simulink model "boostObserver_old"  (R2020a)
settings: Solver=VariableStepAuto  StartTime=0.0  StopTime=3.2  FixedStep=0.0005  MaxStep=9e-06  RelTol=1e-03  EnableMultiTasking=on
InitFcn:
  | kp=0.01;
  | ki=0.01;
  | 
  | k=2;
  | em=100000000;
  | GE=1/em;
  | GU=k*ki/GE;
  | GCE=k*kp/GU;
model workspace (MAT data in the model file):
  time = 0.8
values from neighbouring files (symbols this model uses):
  A1 = obj.boostConverter.A1    [BoostController.m]    (also in BoostConverter.m = [-obj.R/obj.L 0;0 -1/(obj.Ro*obj.C)]; BuckBoostConverter.m = [-obj.R/obj.L 0;0 -1/(obj.Ro*obj.C)]; obsmc.m = Asigma{1,1}; workspace_atual.mat = [-16.4  0; 0  -3.50877192982])
  A2 = obj.boostConverter.A2    [BoostController.m]    (also in BoostConverter.m = [-obj.R/obj.L -1/obj.L;1/obj.C -1/(obj.Ro*obj.C)]; BuckBoostConverter.m = [-obj.R/obj.L 1/obj.L;-1/obj.C -1/(obj.Ro*obj.C)]; obsmc.m = Asigma{1,2}; workspace_atual.mat = [-16.4  -200; 350.877192982  -3.50877192982])
  AlarmDeadTime = 0.50    (= 0.5)    [BoostFaultSimulation.m]    (also in workspace_atual.mat; workspace_certo.mat)
  B1 = obj.boostConverter.B1    [BoostController.m]    (also in BoostConverter.m = [1/obj.L;0]; BuckBoostConverter.m = [1/obj.L;0]; obsmc.m = Bsigma{1,1}; workspace_atual.mat = [200 0])
  boost_parameters = [obj.Ro,obj.R,obj.L,obj.C,obj.u]'    [BoostConverter.m]    (also in BuckBoostConverter.m; boostResults2Latex.m = boost.parameters(); workspace_atual.mat = [100 0.082 0.005 0.00285 190]; workspace_certo.mat = [100 0.082 0.005 0.00285 190])
  C = 1e-3    (= 0.001)    [boostResults2Latex.m]
  CiL = [0 1]    [workspace_atual.mat]    (also in workspace_certo.mat)
  Cmatrix = [1  0; 0  1]    [workspace_atual.mat]    (also in workspace_certo.mat)
  CVc = [1 0]    [workspace_atual.mat]    (also in workspace_certo.mat)
  D1 = [1  0; 0  1]    [workspace_atual.mat]    (also in workspace_certo.mat)
  FaultClass = 0    [BoostFaultSimulation.m]    (also in workspace_atual.mat = 1; workspace_certo.mat = 1)
  iLFaultSwitch = 0    [BoostFaultSimulation.m]    (also in workspace_atual.mat; workspace_certo.mat)
  iLFaultTime = 1.70    (= 1.7)    [BoostFaultSimulation.m]    (also in workspace_atual.mat; workspace_certo.mat)
  iLGainFaultFactor = 15    [BoostFaultSimulation.m]    (also in workspace_atual.mat; workspace_certo.mat)
  iLNoiseFaultSwitch = 0    [BoostFaultSimulation.m]    (also in workspace_atual.mat; workspace_certo.mat)
  iLNoiseTime = 1.70    (= 1.7)    [BoostFaultSimulation.m]    (also in workspace_atual.mat; workspace_certo.mat)
  Jth = 2000    [workspace_atual.mat]    (also in workspace_certo.mat)
  L = 1e-3    (= 0.001)    [boostResults2Latex.m]    (also in obsmc.m = sdpvar(3,1,'full'))
  LoadAddResistor = obj.LoadAddFactor*obj.Ro    [BoostFaultSimulation.m]    (also in workspace_atual.mat = 30; workspace_certo.mat = 30)
  LoadAddSignalSwitch = 1    [BoostFaultSimulation.m]    (also in workspace_atual.mat; workspace_certo.mat)
  LoadAddSwitch = 0    [BoostFaultSimulation.m]    (also in workspace_atual.mat; workspace_certo.mat)
  LoadAddTime = 0.90    (= 0.9)    [BoostFaultSimulation.m]    (also in workspace_atual.mat; workspace_certo.mat)
  LoadRemoveResistor = obj.Ro*(1-obj.LoadRemoveFactor)/(obj.LoadRemoveFactor)    [BoostFaultSimulation.m]    (also in workspace_atual.mat = 233.333333333; workspace_certo.mat = 233.333333333)
  LoadRemoveSignalSwitch = 1    [BoostFaultSimulation.m]    (also in workspace_atual.mat; workspace_certo.mat)
  LoadRemoveSwitch = 0    [BoostFaultSimulation.m]    (also in workspace_atual.mat; workspace_certo.mat)
  LoadRemoveTime = 0.90    (= 0.9)    [BoostFaultSimulation.m]    (also in workspace_atual.mat; workspace_certo.mat)
  LobsiL = [1737913.15707 66180.0912281]    [workspace_atual.mat]    (also in workspace_certo.mat)
  LobsVc = [61200 1]    [workspace_atual.mat]    (also in workspace_certo.mat)
  ObsEp = 70    [workspace_atual.mat]    (also in workspace_certo.mat)
  R = 0.1    [boostResults2Latex.m]    (also in workspace_atual.mat = 0.082; workspace_certo.mat = 0.082)
  ReconfigDelay = 0    [BoostFaultSimulation.m]    (also in workspace_atual.mat = 0.2; workspace_certo.mat = 0.2)
  ReconfigSwitch = 0    [BoostFaultSimulation.m]    (also in workspace_atual.mat; workspace_certo.mat)
  ReconfigTime = 1.707    [BoostFaultSimulation.m]    (also in workspace_atual.mat; workspace_certo.mat)
  rho = 5    [workspace_atual.mat]    (also in workspace_certo.mat)
  RMSfrequency = 47.61    [BoostFaultSimulation.m]    (also in workspace_atual.mat; workspace_certo.mat)
  Ro = 100    [BoostFaultSimulation.m]    (also in boostResults2Latex.m = 10; workspace_atual.mat; workspace_certo.mat)
  Smep = 80    [workspace_atual.mat]    (also in workspace_certo.mat)
  SourceAddSignalSwitch = 1    [BoostFaultSimulation.m]    (also in workspace_atual.mat; workspace_certo.mat)
  SourceAddSwitch = 0    [BoostFaultSimulation.m]    (also in workspace_atual.mat; workspace_certo.mat)
  SourceAddTime = 0.90    (= 0.9)    [BoostFaultSimulation.m]    (also in workspace_atual.mat; workspace_certo.mat)
  SourceAddVoltage = obj.SourceAddFactor*obj.u    [BoostFaultSimulation.m]    (also in workspace_atual.mat = 19; workspace_certo.mat = 19)
  SourceRemoveSignalSwitch = 1    [BoostFaultSimulation.m]    (also in workspace_atual.mat; workspace_certo.mat)
  SourceRemoveSwitch = 0    [BoostFaultSimulation.m]    (also in workspace_atual.mat; workspace_certo.mat)
  SourceRemoveTime = 0.90    (= 0.9)    [BoostFaultSimulation.m]    (also in workspace_atual.mat; workspace_certo.mat)
  SourceRemoveVoltage = obj.SourceRemoveFactor*obj.u    [BoostFaultSimulation.m]    (also in workspace_atual.mat = 19; workspace_certo.mat = 19)
  ueq = 0.5    [workspace_atual.mat]    (also in workspace_certo.mat)
  VcFaultSwitch = 0    [BoostFaultSimulation.m]    (also in workspace_atual.mat; workspace_certo.mat)
  VcFaultTime = 1.70    (= 1.7)    [BoostFaultSimulation.m]    (also in workspace_atual.mat; workspace_certo.mat)
  VcGainFaultFactor = 15    [BoostFaultSimulation.m]    (also in workspace_atual.mat; workspace_certo.mat)
  VcNoiseFaultSwitch = 0    [BoostFaultSimulation.m]    (also in workspace_atual.mat; workspace_certo.mat)
  VcNoiseTime = 1.70    (= 1.7)    [BoostFaultSimulation.m]    (also in workspace_atual.mat; workspace_certo.mat)
  ve = 380    [BoostFaultSimulation.m]    (also in boostResults2Latex.m = 100; workspace_atual.mat; workspace_certo.mat)
  x_e = [ie;ve]    [BoostConverter.m]    (also in BuckBoostConverter.m)
  xe = obj.boostConverter.equilibriumstate(ve)    [BoostController.m]    (also in workspace_atual.mat = [7.62509288104 380]; workspace_certo.mat = [7.62509288104 380])
undefined symbols (not defined in the file or in its folder): Atilde1, Atilde2, Ctilde1, Dtilde1, Dtilde2, F, G, MAXnet, MINnet
libraries: neural x74, powerlib x70, dspstat3 x16, simulink x9, powerlib_meascontrol x7, dspmtrx3 x7, dspmathops x3
(part 1 of 7)
settings Model: SimulationMode=accelerator  Creator=d13go  LastModifiedBy=d13go
settings SolverCC: MaxConsecutiveZCs=10000  ZeroCrossAlgorithm=Adaptive  DecoupledContinuousIntegration=on  MinimalZcImpactIntegration=on
settings DataIOCC: SaveFinalState=on  SaveState=on  LoggingToFile=on
settings OptimizationCC: DefaultParameterBehavior=Inlined  UseDivisionForNetSlopeComputation=on  GainParamInheritBuiltInType=on  UseFloatMulNetSlope=on  InlineInvariantSignals=on  EfficientFloat2IntCast=on  LifeSpan=1
settings DebuggingCC: ReadBeforeWriteMsg=DisableAll  WriteAfterWriteMsg=DisableAll  WriteAfterReadMsg=DisableAll  AlgebraicLoopMsg=error  MaxConsecutiveZCsMsg=warning  MaskedZcDiagnostic=none  IgnoredZcDiagnostic=none  MultiTaskDSMMsg=none  SFUnexpectedBacktrackingDiag=warning  SFNoUnconditionalDefaultTransitionDiag=warning  ArithmeticOperatorsInVariantConditions=warning
settings HardwareCC: ProdLongLongMode=on
settings ModelReferenceCC: UpdateModelReferenceTargets=IfOutOfDate
settings SFSimCC: SFSimEcho=off  SimUseLocalCustomCode=off  MATLABDynamicMemAlloc=off  CustomCodeUndefinedFunction=UseInterfaceOnly
settings RTWCC: GenerateReport=on  RTWUseLocalCustomCode=off  LaunchReport=on
settings CodeAppCC: ForceParamTrailComments=on
settings GRTTargetCC: TargetLangStandard=C89/C90 (ANSI)  CombineSignalStateStructs=on  MatFileLogging=off  SupportVariableSizeSignals=on
settings ConfigComp: CovMetricSettings=dw  CovHtmlReporting=on  CovSaveCumulativeToWorkspaceVar=on  CovSaveSingleToWorkspaceVar=on  CovExternalEMLEnable=off
settings SimscapeCC: SimscapeNormalizeSystem=off

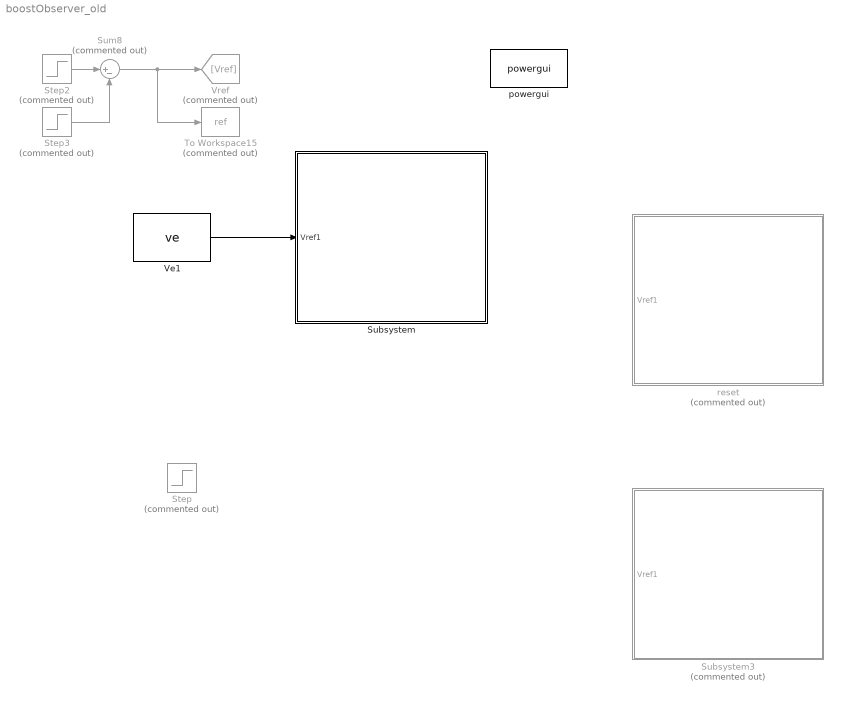
== system boostObserver_old ==
  Step : Step  Commented=on  Time=0.60  Before=380  After=300  SampleTime=0
  Step2 : Step  Commented=on  Time=0  After=100  SampleTime=0
  Step3 : Step  Commented=on  Time=0.4  After=20  SampleTime=0
  Subsystem : Subsystem
  Subsystem3 : Subsystem  Commented=on
  Sum8 : Sum  Commented=on  Inputs=|+-
  To Workspace15 : ToWorkspace  Commented=on  VariableName=ref  SampleTime=-1
  Ve1 : Constant  Value=ve
  Vref : Goto  Commented=on  GotoTag=Vref
  powergui : powerlib/powergui  Priority=1  SimulationMode=Discrete  SampleTime=50e-6  frequency=60  Iterations=50  frequencyindice=0  Pbase=100e6  ErrMax=1e-4  UnitsV=kV  UnitsW=MW  buscounter=0  FunctionMessages=off  echomessages=off  EnableUseOfTLC=off  CurrentSourceSwitches=off  DisableSnubberDevices=off  DisableRonSwitches=off  DisableVfSwitches=off  DisplayEquations=off  AutomaticDiscreteSolvers=off  SolverType=Tustin/Backward Euler (TBE)  Interpol=off  ExternalGateDelay=off  methode=off  Ts=100  x0status=blocks  SPID=on  SwTol=0  HookPort=off  NonlinearTolerance=1e-4  nMaxIteration=100  ContinueOnMaxIteration=off  RestoreLinks=warning  ResistiveCurrentMeasurement=off  Frange=[0:2:500]  Ylog=off  Xlog=on  ShowGrid=off  save=off  variable=ZData  structure=0  ZoomFFT=off  StartTime=0.0  cycles=1  DisplayStyle=1  fundamental=60  FreqAxis=off  MaxFrequency=1000  frequencyindicesteady=1  RmsSteady=1  display=off
  reset : Subsystem  Commented=on
  wires:
  Step2/1 -> Sum8/1
  Step3/1 -> Sum8/2
  Sum8/1 -> To Workspace15/1, Vref/1
  Ve1/1 -> Subsystem/1(Vref1)

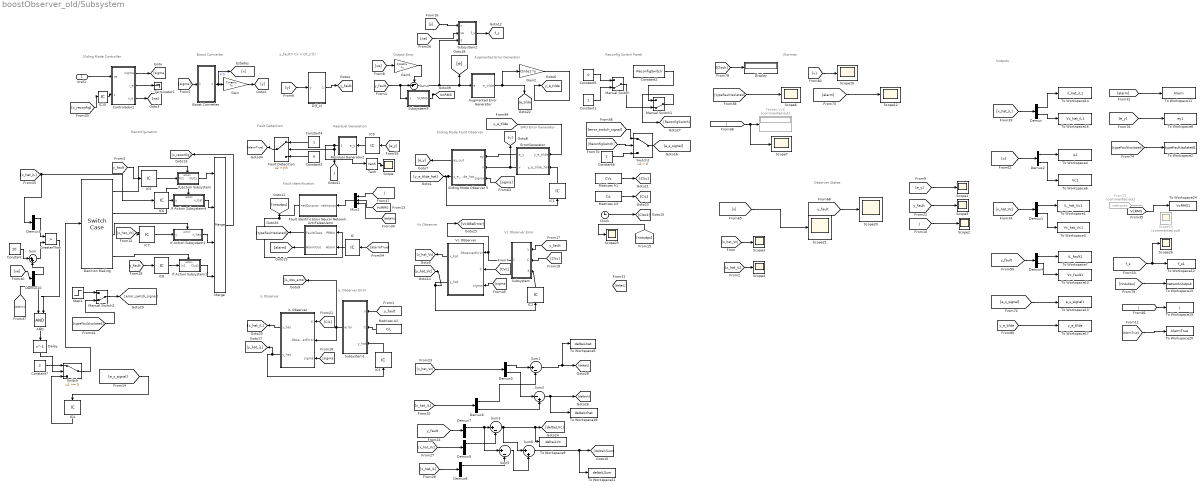
== system boostObserver_old/Subsystem ==
  note: Reconfiguration
  note: Sliding Mode Controller
  note: Boost Converter
  note: Vc Observer
  note: y_fault= Cx + Df_s'(t)
  note: Output Error
  note: Augmented Error Generator
  note: Sliding Mode
      | Fault Observer
  note: SMO Error
      | Generator
  note: Residual Generation
  note: Fault identification
  note: Reconfig Switch Panel
  note: iL Observer
  note: Vc Observer Error
  note: iL Observer Error
  note: Observer States
  note: Outputs
  note: Alarmes
  note: Fault Detection
  Vref1 : Inport
  AND : Logic  IconShape=distinctive  AllPortsSameDT=off  OutDataTypeStr=boolean
  AntiFalseAlarm : Subsystem
  Augmented Error Generator : Subsystem
  Boost Converter : Subsystem
  Clock : Clock
  Constant : Constant  Value=20
  Constant1 : Constant
  Constant2 : Constant  Value=ReconfigSwitch
  Constant3 : Constant  Value=0
  Constant4 : Constant
  Constant5 : Constant  Value=0
  Constant6 : Constant
  Constant7 : Constant  Value=2
  Controlador1 : Subsystem
  D(f_s) : Subsystem
  Decition Making : SwitchCase  CaseConditions={[1,6],[2,3],[4,5]}
  Delay : Delay  DelayLength=1
  Demux{,1..10} (11 alike) : Demux  Outputs=2
  Display : Display
  ErrorGenerator : Subsystem
  Fault Detecition : Switch  Criteria=u2 > Threshold  Threshold=Jth  ZeroCross=off
  Fault Identification Neural Netowrk : Subsystem
  From71 : From  Commented=on  GotoTag=netInputs  TagVisibility=global
  Gain : Gain  Gain=Cmatrix  Multiplication=Matrix(K*u)
  Gain1 : Gain  Gain=Cmatrix  Multiplication=Matrix(K*u)
  Gain2 : Gain  Gain=Ctilde1  Multiplication=Matrix(K*u)
  GreaterThan : RelationalOperator  Operator=>  OutDataTypeStr=boolean  RndMeth=Simplest
  IC : InitialCondition  Value=0
  IC{1,5..10} (7 alike) : InitialCondition  Value=[0;0]
  IC2 : InitialCondition  Value=0
  IC3 : InitialCondition  Value=0
  IC4 : InitialCondition
  If Action Subsystem : Subsystem  TreatAsAtomicUnit=on
  If Action Subsystem1 : Subsystem  TreatAsAtomicUnit=on
  If Action Subsystem2 : Subsystem  TreatAsAtomicUnit=on
  If Action Subsystem4 : Subsystem  TreatAsAtomicUnit=on
  Manual Switch : ManualSwitch  CurrentSetting=0
  Manual Switch1 : ManualSwitch  CurrentSetting=0
  Manual Switch2 : ManualSwitch  CurrentSetting=0
  Matrizes A1 : Constant  Value=CVc  VectorParams1D=off
  Matrizes A2 : Constant  Value=CiL  VectorParams1D=off
  Matrizes A3 : Constant  Value=CiL  VectorParams1D=off
  Merge : Merge  Inputs=4
  Mux2 : Mux  Inputs=3
  Residual Generator2 : Subsystem
  Scope{,1..7,10,12,20..21,25..26} (14 alike) : Scope
  Scope15 : Scope  Commented=on
  Sliding Mode Observer 5 : Subsystem
  Step1 : Step  Time=ReconfigTime  Before=1  After=FaultClass  SampleTime=0
  Subsystem : Subsystem
  Subsystem1 : Subsystem
  Subsystem2 : Subsystem
  Subsystem9 : Subsystem
  Sum : Sum  Inputs=|++
  Sum1 : Sum  Inputs=|+-
  Sum2 : Sum  Inputs=|-+
  Sum3 : Sum  Inputs=|+-
  Sum4 : Sum  Inputs=-+|
  Sum5 : Sum  Inputs=|+-
  Sum6 : Sum  Inputs=|++
  Switch : Switch
  Switch2 : Switch  Criteria=u2 > Threshold
  Tanh : Trigonometry  Operator=tanh
  Tensão Vc6 : Display  Commented=on
  Terminator1 : Terminator
  To Workspace1 : ToWorkspace  VariableName=iL_hat_Vc1  SaveFormat=Timeseries  SampleTime=-1
  To Workspace10 : ToWorkspace  VariableName=Vc_fault1  SaveFormat=Timeseries  SampleTime=-1
  To Workspace11 : ToWorkspace  VariableName=Alarm  SaveFormat=Timeseries  SampleTime=-1
  To Workspace12 : ToWorkspace  VariableName=f_s1  SaveFormat=Timeseries  SampleTime=-1
  To Workspace13 : ToWorkspace  VariableName=e_s_signal1  SaveFormat=Timeseries  SampleTime=-1
  To Workspace14 : ToWorkspace  VariableName=il_hat_iL1  SaveFormat=Timeseries  SampleTime=-1
  To Workspace15 : ToWorkspace  VariableName=networkOutput  SaveFormat=Timeseries  SampleTime=-1
  To Workspace16 : ToWorkspace  VariableName=Vc_hat_iL1  SaveFormat=Timeseries  SampleTime=-1
  To Workspace17 : ToWorkspace  VariableName=y_e_tilde  SaveFormat=Timeseries  SampleTime=-1
  To Workspace18 : ToWorkspace  VariableName=deltaVchat  SaveFormat=Timeseries  SampleTime=-1
  To Workspace19 : ToWorkspace  VariableName=J  SaveFormat=Timeseries  SampleTime=-1
  To Workspace2 : ToWorkspace  VariableName=typeFaultIsolated1  SaveFormat=Timeseries  SampleTime=-1
  To Workspace20 : ToWorkspace  VariableName=AlarmTrue  SaveFormat=Timeseries  SampleTime=-1
  To Workspace21 : ToWorkspace  VariableName=deltaiLSum  SaveFormat=Timeseries  SampleTime=-1
  To Workspace24 : ToWorkspace  VariableName=VcRMS1  SaveFormat=Timeseries  SampleTime=-1
  To Workspace3 : ToWorkspace  VariableName=Vc_hat_Vc1  SaveFormat=Timeseries  SampleTime=-1
  To Workspace4 : ToWorkspace  VariableName=iL1  SaveFormat=Timeseries  SampleTime=-1
  To Workspace5 : ToWorkspace  VariableName=deltaiLhat  SaveFormat=Timeseries  SampleTime=-1
  To Workspace6 : ToWorkspace  VariableName=Vc1  SaveFormat=Timeseries  SampleTime=-1
  To Workspace7 : ToWorkspace  VariableName=iL_fault1  SaveFormat=Timeseries  SampleTime=-1
  To Workspace8 : ToWorkspace  VariableName=ey1  SaveFormat=Timeseries  SampleTime=-1
  To Workspace9 : ToWorkspace  VariableName=deltaiLVc  SaveFormat=Timeseries  SampleTime=-1
  Vc OBserver : Subsystem
  iL Observer : Subsystem
  tag scope: J=global, VcRMS=global, f_s=global, y_e_tilde=global, y_fault=global
  wires:
  Controlador1/2(i_e) -> Terminator1/1
  Vref1/1 -> Controlador1/1(ve)
  Controlador1/3(x_e) -> [xe]
  Controlador1/1(sigma) -> [sigma]
  Boost Converter/1(x) -> [x], Gain/1  "x(t)"
  [sigma] -> Vc OBserver/3(sigma)
  D(f_s)/1(y_fault) -> [y_fault]
  Sum4/1 -> Subsystem2/3(y_fault), [e], Augmented Error Generator/1(e)
  Augmented Error Generator/1(e_tilde) -> [e_tilde], Gain2/1
  [y_e_tilde] -> ErrorGenerator/1(y_e_tilde)
  [e_y] -> Scope1/1
  Gain2/1 -> [y_e_tilde]
  [J] -> Scope2/1
  Mux2/1 -> Fault Identification Neural Netowrk/1(netInputs)
  [J] -> Mux2/1
  Subsystem9/1(VcRMS) -> [VcRMS]
  [typeFaultIsolated] -> Manual Switch2/2
  Manual Switch2/1 -> [error_switch_signal]
  Decition Making/1 -> If Action Subsystem/Action
  If Action Subsystem/1(Out1) -> Merge/1
  Decition Making/3 -> If Action Subsystem2/Action
  [y_fault] -> Subsystem/1(y)
  Clock/1 -> [Clock]
  [ReconfigSwitch] -> Switch2/2
  Switch2/1 -> [e_s_signal]
  Manual Switch/1 -> Manual Switch1/2
  Constant1/1 -> Manual Switch/2
  Constant2/1 -> Manual Switch1/1
  Constant5/1 -> Manual Switch/1
  Constant6/1 -> Switch2/3
  Manual Switch1/1 -> [ReconfigSwitch]
  [error_switch_signal] -> Switch2/1
  Decition Making/2 -> If Action Subsystem4/Action
  Matrizes A2/1 -> Subsystem1/2(C)
  iL Observer/1(x_hat) -> [x_hat_iL]
  Matrizes A1/1 -> [CVc]
  [CVc] -> Subsystem/2(C)
  Matrizes A3/1 -> [CiL]
  [CiL] -> iL Observer/1(C)
  [y_fault] -> IC8/1
  Step1/1 -> Manual Switch2/1
  [x_hat_iL] -> Scope4/1
  [y_fault] -> Scope5/1
  [sigma] -> Boost Converter/1(sigma)
  [alarmTrue] -> IC/1
  AntiFalseAlarm/1(FaultClass) -> [typeFaultIsolated]
  [x_hat_iL] -> Demux/1
  Demux/1 -> To Workspace14/1
  Demux1/2 -> To Workspace3/1
  [J] -> Tensão Vc6/1, Scope7/1
  [y_fault] -> Demux4/1
  Demux4/2 -> To Workspace10/1
  Demux2/2 -> To Workspace6/1
  [typeFaultIsolated] -> Scope6/1
  [alarm] -> Scope12/1
  [e_y] -> To Workspace8/1
  [f_s] -> Scope26/1, To Workspace12/1
  [y_fault] -> Scope20/1
  [alarm] -> To Workspace11/1
  [e_s_signal] -> To Workspace13/1
  Demux2/1 -> To Workspace4/1
  Demux1/1 -> To Workspace1/1
  [x] -> Scope21/1
  From71/1 -> ?
  [x] -> Demux2/1
  [typeFaultIsolated] -> To Workspace2/1
  [Clock] -> Display/1
  Demux/2 -> To Workspace16/1
  Demux4/1 -> To Workspace7/1
  [x_hat_Vc] -> Demux1/1
  [nnoutpu] -> To Workspace15/1
  [y_e_tilde] -> To Workspace17/1
  [J] -> To Workspace19/1
  Constant4/1 -> Fault Detecition/1
  Constant3/1 -> Fault Detecition/3
  Fault Detecition/1 -> [alarmTrue]
  [v] -> Scope10/1
  [y_fault] -> Subsystem1/1(y)
  Vc OBserver/2(y_hat) -> IC2/1, [y_hat_Vc]
  [y_fault] -> Subsystem9/1(x), Sum4/2
  Gain/1 -> [y]
  [y] -> D(f_s)/1(y)
  [xe] -> Gain1/1
  Gain1/1 -> Sum4/1
  ErrorGenerator/1(e_y) -> Sliding Mode Observer 5/1(ey)
  ErrorGenerator/2(v) -> Sliding Mode Observer 5/2(v), [v]
  [sigma] -> Sliding Mode Observer 5/3(sigma)
  Sliding Mode Observer 5/2(y_e_tilde_hat) -> IC1/1, [y_e_tilde_hat]
  Sliding Mode Observer 5/1(ey_out) -> [e_y]
  IC/1 -> AntiFalseAlarm/2(Alarm)
  Subsystem/1(error) -> [VcOBsErrror], Vc OBserver/1(ObserverError)
  Vc OBserver/1(x_hat) -> [x_hat_Vc]
  [sigma] -> iL Observer/3(sigma)
  Subsystem1/1(error) -> iL Observer/2(ObserverError), [iL_obs_error]
  [CVc] -> Vc OBserver/2(C)
  iL Observer/2(y_hat) -> IC3/1, [y_hat_iL]
  IC1/1 -> ErrorGenerator/2(y_e_tilde_hat)
  IC2/1 -> Subsystem/3(y_hat)
  IC3/1 -> Subsystem1/3(y_hat)
  IC5/1 -> If Action Subsystem/1(In1)
  [y_fault] -> IC5/1
  [x_hat_iL] -> Demux3/1, IC6/1
  IC7/1 -> If Action Subsystem2/1(y)
  [x_hat_Vc] -> IC7/1
  IC8/1 -> If Action Subsystem1/1(In1)
  [e_y] -> IC9/1
  IC9/1 -> Residual Generator2/1(e_y)
  [x_reconfig] -> IC10/1
  IC10/1 -> Controlador1/2(x)
  AntiFalseAlarm/2(AlarmOut) -> [alarm]
  [alarmTrue] -> To Workspace20/1
  Decition Making/4 -> If Action Subsystem1/Action
  IC6/1 -> If Action Subsystem4/1(y)
  If Action Subsystem4/1(x_hat) -> Merge/2
  [x_hat_Vc] -> Demux5/1
  [x_hat_iL] -> Demux6/1
  Demux5/1 -> Sum1/1
  Demux6/1 -> Sum1/2
  Demux5/2 -> Sum2/1
  Demux6/2 -> Sum2/2
  Sum2/1 -> To Workspace18/1, [deltaVc]
  Fault Identification Neural Netowrk/1(netOutputs) -> AntiFalseAlarm/1(PRNN), [nnoutpu]
  Sum1/1 -> To Workspace5/1, [deltaiL]
  If Action Subsystem2/1(x_hat) -> Merge/3
  If Action Subsystem1/1(Out1) -> Merge/4
  Merge/1 -> [x_reconfig]
  [y_fault] -> Demux7/1
  Demux7/1 -> Sum5/1, Sum3/1
  [x_hat_Vc] -> Demux9/1
  [x_hat_iL] -> Demux8/1
  Demux9/1 -> Sum3/2
  Demux8/1 -> Sum5/2
  [nnoutpu] -> Scope25/1
  [xe] -> Subsystem2/2(xe)
  Subsystem2/1(f_s) -> [f_s]
  [y] -> Subsystem2/1(x)
  [x_hat_Vc] -> Scope3/1
  Sum3/1 -> To Workspace9/1, [deltaiLVc], Sum6/1
  Sum5/1 -> Sum6/2
  Sum6/1 -> To Workspace21/1, [deltaiLSum]
  [VcRMS] -> To Workspace24/1
  [VcRMS] -> Mux2/2
  [deltaVc] -> Mux2/3
  Residual Generator2/1(RMS) -> Tanh/1, Fault Detecition/2, [J]
  Tanh/1 -> Scope/1
  IC4/1 -> Switch/3
  Constant7/1 -> Switch/1
  Switch/1 -> Decition Making/1
  [e_s_signal] -> IC4/1
  GreaterThan/1 -> AND/2
  AND/1 -> Delay/1
  [alarm] -> AND/1
  Demux3/1 -> GreaterThan/1
  Delay/1 -> Switch/2
  Constant/1 -> Sum/1
  [xe] -> Demux10/1
  Sum/1 -> GreaterThan/2
  Demux10/1 -> Sum/2

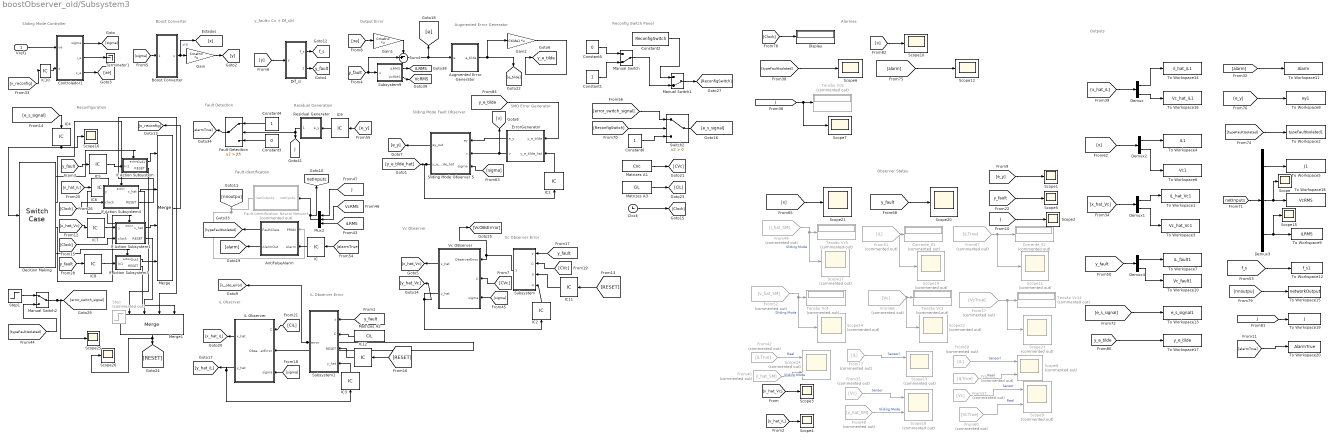
== system boostObserver_old/Subsystem3 ==
  note: Reconfiguration
  note: Sliding Mode Controller
  note: Boost Converter
  note: Vc Observer
  note: y_fault= Cx + Df_s(t)
  note: Output Error
  note: Augmented Error Generator
  note: Sliding Mode
      | Fault Observer
  note: SMO Error
      | Generator
  note: Residual Generation
  note: Fault identification
  note: Reconfig Switch Panel
  note: iL Observer
  note: Vc Observer Error
  note: iL Observer Error
  note: Observer States
  note: Outputs
  note: Alarmes
  note: Fault Detection
  Vref1 : Inport
  AntiFalseAlarm : Subsystem
  Augmented Error Generator : Subsystem
  Boost Converter : Subsystem
  Clock : Clock
  Constant1 : Constant
  Constant2 : Constant  Value=ReconfigSwitch
  Constant3 : Constant  Value=0
  Constant4 : Constant
  Constant5 : Constant  Value=0
  Constant6 : Constant
  Controlador1 : Subsystem
  Corrente_Il1 : Display  Commented=on
  Corrente_Il2 : Display  Commented=on
  D(f_s) : Subsystem
  Decition Making : SwitchCase  CaseConditions={[1,6],[2,3],[4,5]}
  Demux{,1..2,4} (4 alike) : Demux  Outputs=2
  Demux3 : Demux  Outputs=3
  Display : Display
  ErrorGenerator : Subsystem
  Fault Detecition : Switch  Criteria=u2 > Threshold  Threshold=Jth  ZeroCross=off
  Fault Identification Neural Netowrk : Subsystem  Commented=on
  From35 : From  Commented=on  GotoTag=Vc
  From37 : From  Commented=on  GotoTag=VcTrue
  From40 : From  Commented=on  GotoTag=i_hat_SM  TagVisibility=global
  From42 : From  Commented=on  GotoTag=iLTrue
  From48 : From  Commented=on  GotoTag=v_hat_SM  TagVisibility=global
  From49 : From  Commented=on  GotoTag=i_hat_SM  TagVisibility=global
  From51 : From  Commented=on  GotoTag=iL
  From52 : From  Commented=on  GotoTag=v_hat_SM  TagVisibility=global
  From57 : From  Commented=on  GotoTag=Vc
  From60 : From  Commented=on  GotoTag=VcTrue
  From66 : From  Commented=on  GotoTag=Vc
  From67 : From  Commented=on  GotoTag=iLTrue
  From69 : From  Commented=on  GotoTag=iL
  From73 : From  Commented=on  GotoTag=iLTrue
  From77 : From  Commented=on  GotoTag=iL
  Gain : Gain  Gain=Cmatrix  Multiplication=Matrix(K*u)
  Gain1 : Gain  Gain=Cmatrix  Multiplication=Matrix(K*u)
  Gain2 : Gain  Gain=Ctilde1  Multiplication=Matrix(K*u)
  IC{,2..3,11..12} (5 alike) : InitialCondition  Value=0
  IC{1,5..10} (7 alike) : InitialCondition  Value=[0;0]
  IC4 : InitialCondition
  If Action Subsystem : Subsystem  TreatAsAtomicUnit=on
  If Action Subsystem1 : Subsystem  TreatAsAtomicUnit=on
  If Action Subsystem3 : Subsystem  TreatAsAtomicUnit=on
  If Action Subsystem4 : Subsystem  TreatAsAtomicUnit=on
  Manual Switch : ManualSwitch  CurrentSetting=0
  Manual Switch1 : ManualSwitch  CurrentSetting=0
  Manual Switch2 : ManualSwitch
  Matrizes A1 : Constant  Value=CVc  VectorParams1D=off
  Matrizes A2 : Constant  Value=CiL  VectorParams1D=off
  Matrizes A3 : Constant  Value=CiL  VectorParams1D=off
  Merge : Merge  Inputs=4
  Merge1 : Merge  Inputs=4
  Mux2 : Mux  Inputs=3
  Residual Generator : Subsystem
  Scope{,1..7,10,12,15..16,20..21,25..26} (16 alike) : Scope
  Scope{11,14,17,19,22..23} (6 alike) : Scope  Commented=on
  Scope{8..9,13,18,24} (5 alike) : Scope  Commented=on  NumInputPorts=2
  Sliding Mode Observer 5 : Subsystem
  Step : Step  Commented=on  Time=1.61  Before=1  After=2  SampleTime=0
  Step1 : Step  Time=ReconfigTime  Before=1  After=FaultClass  SampleTime=0
  Subsystem : Subsystem
  Subsystem1 : Subsystem
  Subsystem9 : Subsystem
  Sum4 : Sum  Inputs=-+|
  Switch2 : Switch  Criteria=u2 > Threshold
  Tensão Vc{1,4..6,14} (5 alike) : Display  Commented=on
  Terminator1 : Terminator
  To Workspace1 : ToWorkspace  VariableName=iL_hat_Vc1  SaveFormat=Timeseries  SampleTime=-1
  To Workspace10 : ToWorkspace  VariableName=Vc_fault1  SaveFormat=Timeseries  SampleTime=-1
  To Workspace11 : ToWorkspace  VariableName=Alarm  SaveFormat=Timeseries  SampleTime=-1
  To Workspace12 : ToWorkspace  VariableName=f_s1  SaveFormat=Timeseries  SampleTime=-1
  To Workspace13 : ToWorkspace  VariableName=e_s_signal1  SaveFormat=Timeseries  SampleTime=-1
  To Workspace14 : ToWorkspace  VariableName=il_hat_iL1  SaveFormat=Timeseries  SampleTime=-1
  To Workspace15 : ToWorkspace  VariableName=networkOutput  SaveFormat=Timeseries  SampleTime=-1
  To Workspace16 : ToWorkspace  VariableName=Vc_hat_iL1  SaveFormat=Timeseries  SampleTime=-1
  To Workspace17 : ToWorkspace  VariableName=y_e_tilde  SaveFormat=Timeseries  SampleTime=-1
  To Workspace18 : ToWorkspace  VariableName=VcRMS  SaveFormat=Timeseries  SampleTime=-1
  To Workspace19 : ToWorkspace  VariableName=J  SaveFormat=Timeseries  SampleTime=-1
  To Workspace2 : ToWorkspace  VariableName=typeFaultIsolated1  SaveFormat=Timeseries  SampleTime=-1
  To Workspace20 : ToWorkspace  VariableName=AlarmTrue  SaveFormat=Timeseries  SampleTime=-1
  To Workspace3 : ToWorkspace  VariableName=Vc_hat_Vc1  SaveFormat=Timeseries  SampleTime=-1
  To Workspace4 : ToWorkspace  VariableName=iL1  SaveFormat=Timeseries  SampleTime=-1
  To Workspace5 : ToWorkspace  VariableName=J1  SaveFormat=Timeseries  SampleTime=-1
  To Workspace6 : ToWorkspace  VariableName=Vc1  SaveFormat=Timeseries  SampleTime=-1
  To Workspace7 : ToWorkspace  VariableName=iL_fault1  SaveFormat=Timeseries  SampleTime=-1
  To Workspace8 : ToWorkspace  VariableName=ey1  SaveFormat=Timeseries  SampleTime=-1
  To Workspace9 : ToWorkspace  VariableName=iLRMS  SaveFormat=Timeseries  SampleTime=-1
  Vc OBserver : Subsystem
  iL Observer : Subsystem
  tag scope: J=global, VcRMS=global, f_s=global, iLRMS=global, netInputs=global, y_e_tilde=global, y_fault=global
  wires:
  Controlador1/2(i_e) -> Terminator1/1
  Vref1/1 -> Controlador1/1(ve)
  Controlador1/3(x_e) -> [xe]
  Controlador1/1(sigma) -> [sigma]
  Boost Converter/1(x) -> [x], Gain/1  "x(t)"
  [sigma] -> Vc OBserver/3(sigma)
  D(f_s)/1(f_s) -> [f_s]
  D(f_s)/2(y_fault) -> [y_fault]
  Sum4/1 -> [e], Augmented Error Generator/1(e)
  Augmented Error Generator/1(e_tilde) -> [e_tilde], Gain2/1
  [y_e_tilde] -> ErrorGenerator/1(y_e_tilde)
  [e_y] -> Scope1/1
  Gain2/1 -> [y_e_tilde]
  [J] -> Scope2/1
  Mux2/1 -> [netInputs], Fault Identification Neural Netowrk/1(netInputs)
  [VcRMS] -> Mux2/2
  [J] -> Mux2/1
  [iLRMS] -> Mux2/3
  Subsystem9/2(VcRMS) -> [VcRMS]
  Subsystem9/1(iLRMS) -> [iLRMS]
  [typeFaultIsolated] -> Manual Switch2/2
  Manual Switch2/1 -> Scope25/1, [error_switch_signal]
  Decition Making/1 -> If Action Subsystem/Action
  [x_hat_Vc] -> Scope3/1
  If Action Subsystem/1(Out1) -> Merge/1
  Decition Making/3 -> If Action Subsystem1/Action
  Merge/1 -> [x_reconfig]
  [y_fault] -> Subsystem/1(y)
  Clock/1 -> [Clock]
  [ReconfigSwitch] -> Switch2/2
  Switch2/1 -> [e_s_signal]
  Manual Switch/1 -> Manual Switch1/2
  Constant1/1 -> Manual Switch/2
  Constant2/1 -> Manual Switch1/1
  Constant5/1 -> Manual Switch/1
  Constant6/1 -> Switch2/3
  Manual Switch1/1 -> [ReconfigSwitch]
  [error_switch_signal] -> Switch2/1
  [e_s_signal] -> IC4/1
  Decition Making/2 -> If Action Subsystem4/Action
  Matrizes A2/1 -> Subsystem1/2(C)
  iL Observer/1(x_hat) -> [x_hat_iL]
  Matrizes A1/1 -> [CVc]
  [CVc] -> Subsystem/2(C)
  Matrizes A3/1 -> [CiL]
  [CiL] -> iL Observer/1(C)
  [Clock] -> If Action Subsystem4/2(clock)
  [y_fault] -> IC8/1
  Step1/1 -> Manual Switch2/1
  [x_hat_iL] -> Scope4/1
  [y_fault] -> Scope5/1
  [sigma] -> Boost Converter/1(sigma)
  [alarmTrue] -> IC/1
  AntiFalseAlarm/1(FaultClass) -> [typeFaultIsolated]
  Fault Identification Neural Netowrk/1(netOutputs) -> AntiFalseAlarm/1(PRNN), [nnoutpu]
  [x_hat_iL] -> Demux/1
  From51/1 -> Corrente_Il1/1, Scope19/1
  Demux/1 -> To Workspace14/1
  Demux1/2 -> To Workspace3/1
  [J] -> Tensão Vc6/1, Scope7/1
  [y_fault] -> Demux4/1
  From40/1 -> Scope24/2  "Sliding Mode"
  Demux4/2 -> To Workspace10/1
  Demux2/2 -> To Workspace6/1
  From48/1 -> Scope18/2  "Sliding Mode"
  [typeFaultIsolated] -> Scope6/1
  From35/1 -> Scope18/1  "Sensor"
  [alarm] -> Scope12/1
  [e_y] -> To Workspace8/1
  [f_s] -> To Workspace12/1
  [y_fault] -> Scope20/1
  [alarm] -> To Workspace11/1
  [e_s_signal] -> To Workspace13/1
  Demux3/2 -> Scope/1, To Workspace18/1
  Demux2/1 -> To Workspace4/1
  From77/1 -> Scope13/1  "Sensorl"
  Demux1/1 -> To Workspace1/1
  [x] -> Scope21/1
  Demux3/3 -> To Workspace9/1, Scope15/1
  [netInputs] -> Demux3/1
  Demux3/1 -> To Workspace5/1
  [x] -> Demux2/1
  From37/1 -> Tensão Vc14/1, Scope23/1
  From73/1 -> Scope8/2  "Real"
  From52/1 -> Scope14/1, Tensão Vc4/1  "Sliding Mode"
  [typeFaultIsolated] -> To Workspace2/1
  From42/1 -> Scope24/1  "Real"
  From69/1 -> Scope8/1  "Sensorl"
  [Clock] -> Display/1
  From49/1 -> Scope17/1, Tensão Vc5/1  "Sliding Mode"
  From60/1 -> Scope9/2  "Real"
  Demux/2 -> To Workspace16/1
  From57/1 -> Scope9/1  "Sensor"
  Demux4/1 -> To Workspace7/1
  From66/1 -> Scope22/1, Tensão Vc1/1
  [x_hat_Vc] -> Demux1/1
  From67/1 -> Scope11/1, Corrente_Il2/1
  [nnoutpu] -> To Workspace15/1
  [y_e_tilde] -> To Workspace17/1
  [J] -> To Workspace19/1
  Constant4/1 -> Fault Detecition/1
  Constant3/1 -> Fault Detecition/3
  Residual Generator/1(RMS) -> Fault Detecition/2, [J]
  Fault Detecition/1 -> [alarmTrue]
  [v] -> Scope10/1
  [y_fault] -> Subsystem1/1(y)
  Vc OBserver/2(y_hat) -> IC2/1, [y_hat_Vc]
  [y_fault] -> Sum4/2, Subsystem9/1(x)
  Gain/1 -> [y]
  [y] -> D(f_s)/1(y)
  [xe] -> Gain1/1
  Gain1/1 -> Sum4/1
  ErrorGenerator/1(e_y) -> Sliding Mode Observer 5/1(ey)
  ErrorGenerator/2(v) -> Sliding Mode Observer 5/2(v), [v]
  [sigma] -> Sliding Mode Observer 5/3(sigma)
  Sliding Mode Observer 5/2(y_e_tilde_hat) -> IC1/1, [y_e_tilde_hat]
  Sliding Mode Observer 5/1(ey_out) -> [e_y]
  IC/1 -> AntiFalseAlarm/2(Alarm)
  Subsystem/1(error) -> [VcOBsErrror], Vc OBserver/1(ObserverError)
  Vc OBserver/1(x_hat) -> [x_hat_Vc]
  [sigma] -> iL Observer/3(sigma)
  Subsystem1/1(error) -> [iL_obs_error], iL Observer/2(ObserverError)
  [CVc] -> Vc OBserver/2(C)
  iL Observer/2(y_hat) -> IC3/1, [y_hat_iL]
  IC1/1 -> ErrorGenerator/2(y_e_tilde_hat)
  IC2/1 -> Subsystem/4(y_hat)
  IC3/1 -> Subsystem1/4(y_hat)
  IC4/1 -> Decition Making/1, Scope16/1
  IC5/1 -> If Action Subsystem/1(In1)
  [y_fault] -> IC5/1
  [x_hat_iL] -> IC6/1
  IC7/1 -> If Action Subsystem1/1(y)
  [x_hat_Vc] -> IC7/1
  IC8/1 -> If Action Subsystem3/1(In1)
  [e_y] -> IC9/1
  IC9/1 -> Residual Generator/1(e_y)
  [x_reconfig] -> IC10/1
  IC10/1 -> Controlador1/2(x)
  AntiFalseAlarm/2(AlarmOut) -> [alarm]
  [alarmTrue] -> To Workspace20/1
  [Clock] -> If Action Subsystem1/2(clock)
  If Action Subsystem1/1(x_hat) -> Merge/3
  Decition Making/4 -> If Action Subsystem3/Action
  If Action Subsystem3/1(Out1) -> Merge/4
  If Action Subsystem/2(RESET) -> Merge1/1
  If Action Subsystem1/2(RESET) -> Merge1/2
  If Action Subsystem3/2(RESET) -> Merge1/4
  Merge1/1 -> Scope26/1, [RESET]
  [RESET] -> IC11/1
  IC11/1 -> Subsystem/3(RESET)
  IC12/1 -> Subsystem1/3(RESET)
  [RESET] -> IC12/1
  IC6/1 -> If Action Subsystem4/1(y)
  If Action Subsystem4/1(x_hat) -> Merge/2
  If Action Subsystem4/2(RESET) -> Merge1/3

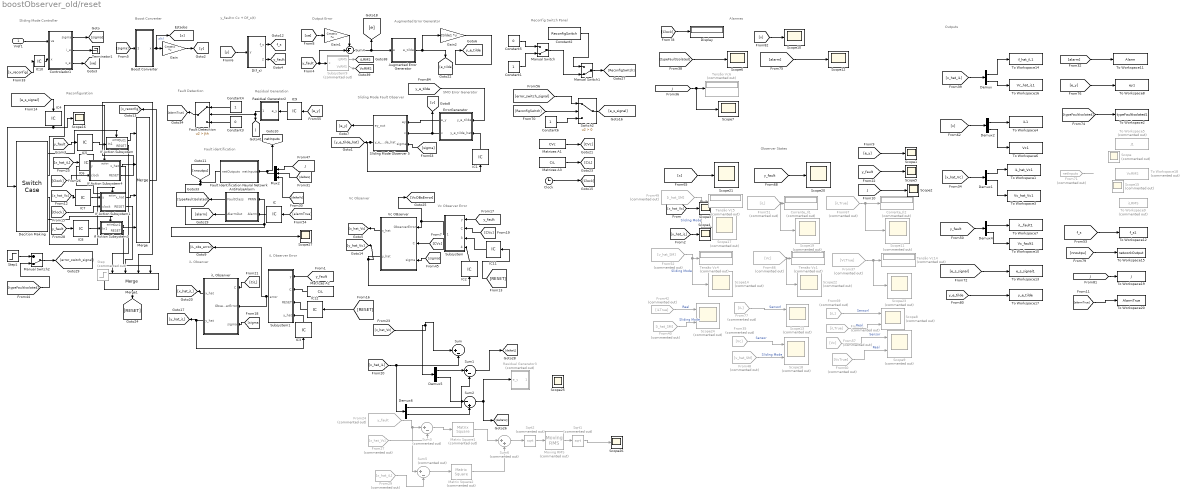
== system boostObserver_old/reset ==
  note: Reconfiguration
  note: Sliding Mode Controller
  note: Boost Converter
  note: Vc Observer
  note: y_fault= Cx + Df_s(t)
  note: Output Error
  note: Augmented Error Generator
  note: Sliding Mode
      | Fault Observer
  note: SMO Error
      | Generator
  note: Residual Generation
  note: Fault identification
  note: Reconfig Switch Panel
  note: iL Observer
  note: Vc Observer Error
  note: iL Observer Error
  note: Observer States
  note: Outputs
  note: Alarmes
  note: Fault Detection
  Vref1 : Inport
  AntiFalseAlarm : Subsystem
  Augmented Error Generator : Subsystem
  Boost Converter : Subsystem
  Clock : Clock
  Constant1 : Constant
  Constant2 : Constant  Value=ReconfigSwitch
  Constant3 : Constant  Value=0
  Constant4 : Constant
  Constant5 : Constant  Value=0
  Constant6 : Constant
  Controlador1 : Subsystem
  Corrente_Il1 : Display  Commented=on
  Corrente_Il2 : Display  Commented=on
  D(f_s) : Subsystem
  Decition Making : SwitchCase  CaseConditions={[1,6],[2,3],[4,5]}
  Demux{,1..2,4..6} (6 alike) : Demux  Outputs=2
  Display : Display
  ErrorGenerator : Subsystem
  Fault Detecition : Switch  Criteria=u2 > Threshold  Threshold=Jth  ZeroCross=off
  Fault Identification Neural Netowrk : Subsystem
  From24 : From  Commented=on  GotoTag=y_fault  TagVisibility=global
  From27 : From  Commented=on  GotoTag=x_hat_Vc
  From29 : From  Commented=on  GotoTag=x_hat_iL
  From35 : From  Commented=on  GotoTag=Vc
  From37 : From  Commented=on  GotoTag=VcTrue
  From40 : From  Commented=on  GotoTag=i_hat_SM  TagVisibility=global
  From42 : From  Commented=on  GotoTag=iLTrue
  From48 : From  Commented=on  GotoTag=v_hat_SM  TagVisibility=global
  From49 : From  Commented=on  GotoTag=i_hat_SM  TagVisibility=global
  From51 : From  Commented=on  GotoTag=iL
  From52 : From  Commented=on  GotoTag=v_hat_SM  TagVisibility=global
  From57 : From  Commented=on  GotoTag=Vc
  From60 : From  Commented=on  GotoTag=VcTrue
  From66 : From  Commented=on  GotoTag=Vc
  From67 : From  Commented=on  GotoTag=iLTrue
  From69 : From  Commented=on  GotoTag=iL
  From71 : From  Commented=on  GotoTag=netInputs  TagVisibility=global
  From73 : From  Commented=on  GotoTag=iLTrue
  From77 : From  Commented=on  GotoTag=iL
  Gain : Gain  Gain=Cmatrix  Multiplication=Matrix(K*u)
  Gain1 : Gain  Gain=Cmatrix  Multiplication=Matrix(K*u)
  Gain2 : Gain  Gain=Ctilde1  Multiplication=Matrix(K*u)
  IC{,2..3,11..12} (5 alike) : InitialCondition  Value=0
  IC{1,5..10} (7 alike) : InitialCondition  Value=[0;0]
  IC4 : InitialCondition
  If Action Subsystem : Subsystem  TreatAsAtomicUnit=on
  If Action Subsystem1 : Subsystem  TreatAsAtomicUnit=on
  If Action Subsystem3 : Subsystem  TreatAsAtomicUnit=on
  If Action Subsystem4 : Subsystem  TreatAsAtomicUnit=on
  Manual Switch : ManualSwitch  CurrentSetting=0
  Manual Switch1 : ManualSwitch  CurrentSetting=0
  Manual Switch2 : ManualSwitch  CurrentSetting=0
  Matrix Square1 : dspmtrx3/Matrix Square  Commented=on  OutMin=[]  OutMax=[]
      settings: SourceProductBaseCode=DS
  Matrix Square2 : dspmtrx3/Matrix Square  Commented=on  OutMin=[]  OutMax=[]
      settings: SourceProductBaseCode=DS
  Matrizes A1 : Constant  Value=CVc  VectorParams1D=off
  Matrizes A2 : Constant  Value=CiL  VectorParams1D=off
  Matrizes A3 : Constant  Value=CiL  VectorParams1D=off
  Merge : Merge  Inputs=4
  Merge1 : Merge  Inputs=4
  Moving RMS : dspstat3/Moving RMS  Commented=on  Method=Sliding window  ForgettingFactorPort=off  SpecifyWindowLength=on  WindowLength=2*RMSfrequency  ForgettingFactor=0.9  SimulateUsing=Code generation
      settings: SourceProductBaseCode=DS
  Mux2 : Mux  Inputs=3
  Residual Generator2 : Subsystem
  Residual Generator3 : Subsystem  Commented=on
  Scope{,11,14..15,17,19,22..23} (8 alike) : Scope  Commented=on
  Scope{1..7,10,12,16,20..21,25..27} (15 alike) : Scope
  Scope{8..9,13,18,24} (5 alike) : Scope  Commented=on  NumInputPorts=2
  Sliding Mode Observer 5 : Subsystem
  Sqrt1 : Sqrt  Commented=on  SaturateOnIntegerOverflow=on
  Sqrt2 : Sqrt  Commented=on  SaturateOnIntegerOverflow=on
  Step : Step  Commented=on  Time=1.61  Before=1  After=2  SampleTime=0
  Step1 : Step  Time=ReconfigTime  Before=1  After=FaultClass  SampleTime=0
  Subsystem : Subsystem
  Subsystem1 : Subsystem
  Subsystem9 : Subsystem  Commented=on
  Sum : Sum  Inputs=|+-
  Sum1 : Sum  Inputs=|+-
  Sum2 : Sum  Inputs=|-+
  Sum3 : Sum  Commented=on  Inputs=|+-
  Sum4 : Sum  Inputs=-+|
  Sum5 : Sum  Commented=on  Inputs=|+-
  Sum6 : Sum  Commented=on  Inputs=|++
  Switch2 : Switch  Criteria=u2 > Threshold
  Tensão Vc{1,4..6,14} (5 alike) : Display  Commented=on
  Terminator1 : Terminator
  To Workspace1 : ToWorkspace  VariableName=iL_hat_Vc1  SaveFormat=Timeseries  SampleTime=-1
  To Workspace10 : ToWorkspace  VariableName=Vc_fault1  SaveFormat=Timeseries  SampleTime=-1
  To Workspace11 : ToWorkspace  VariableName=Alarm  SaveFormat=Timeseries  SampleTime=-1
  To Workspace12 : ToWorkspace  VariableName=f_s1  SaveFormat=Timeseries  SampleTime=-1
  To Workspace13 : ToWorkspace  VariableName=e_s_signal1  SaveFormat=Timeseries  SampleTime=-1
  To Workspace14 : ToWorkspace  VariableName=il_hat_iL1  SaveFormat=Timeseries  SampleTime=-1
  To Workspace15 : ToWorkspace  VariableName=networkOutput  SaveFormat=Timeseries  SampleTime=-1
  To Workspace16 : ToWorkspace  VariableName=Vc_hat_iL1  SaveFormat=Timeseries  SampleTime=-1
  To Workspace17 : ToWorkspace  VariableName=y_e_tilde  SaveFormat=Timeseries  SampleTime=-1
  To Workspace18 : ToWorkspace  Commented=on  VariableName=VcRMS  SaveFormat=Timeseries  SampleTime=-1
  To Workspace19 : ToWorkspace  VariableName=J  SaveFormat=Timeseries  SampleTime=-1
  To Workspace2 : ToWorkspace  VariableName=typeFaultIsolated1  SaveFormat=Timeseries  SampleTime=-1
  To Workspace20 : ToWorkspace  VariableName=AlarmTrue  SaveFormat=Timeseries  SampleTime=-1
  To Workspace3 : ToWorkspace  VariableName=Vc_hat_Vc1  SaveFormat=Timeseries  SampleTime=-1
  To Workspace4 : ToWorkspace  VariableName=iL1  SaveFormat=Timeseries  SampleTime=-1
  To Workspace5 : ToWorkspace  Commented=on  VariableName=J1  SaveFormat=Timeseries  SampleTime=-1
  To Workspace6 : ToWorkspace  VariableName=Vc1  SaveFormat=Timeseries  SampleTime=-1
  To Workspace7 : ToWorkspace  VariableName=iL_fault1  SaveFormat=Timeseries  SampleTime=-1
  To Workspace8 : ToWorkspace  VariableName=ey1  SaveFormat=Timeseries  SampleTime=-1
  To Workspace9 : ToWorkspace  Commented=on  VariableName=iLRMS  SaveFormat=Timeseries  SampleTime=-1
  Vc OBserver : Subsystem
  iL Observer : Subsystem
  tag scope: J=global, VcRMS=global, f_s=global, iLRMS=global, netInputs=global, y_e_tilde=global, y_fault=global
  wires:
  Controlador1/2(i_e) -> Terminator1/1
  Vref1/1 -> Controlador1/1(ve)
  Controlador1/3(x_e) -> [xe]
  Controlador1/1(sigma) -> [sigma]
  Boost Converter/1(x) -> [x], Gain/1  "x(t)"
  [sigma] -> Vc OBserver/3(sigma)
  D(f_s)/1(f_s) -> [f_s]
  D(f_s)/2(y_fault) -> [y_fault]
  Sum4/1 -> [e], Augmented Error Generator/1(e)
  Augmented Error Generator/1(e_tilde) -> [e_tilde], Gain2/1
  [y_e_tilde] -> ErrorGenerator/1(y_e_tilde)
  [e_y] -> Scope1/1
  Gain2/1 -> [y_e_tilde]
  [J] -> Scope2/1
  Mux2/1 -> [netInputs], Fault Identification Neural Netowrk/1(netInputs)
  [J] -> Mux2/1
  Subsystem9/2(VcRMS) -> [VcRMS]
  Subsystem9/1(iLRMS) -> [iLRMS]
  [typeFaultIsolated] -> Manual Switch2/2
  Manual Switch2/1 -> [error_switch_signal]
  Decition Making/1 -> If Action Subsystem/Action
  [x_hat_Vc] -> Scope3/1
  If Action Subsystem/1(Out1) -> Merge/1
  Decition Making/3 -> If Action Subsystem1/Action
  Merge/1 -> [x_reconfig]
  [y_fault] -> Subsystem/1(y)
  Clock/1 -> [Clock]
  [ReconfigSwitch] -> Switch2/2
  Switch2/1 -> [e_s_signal]
  Manual Switch/1 -> Manual Switch1/2
  Constant1/1 -> Manual Switch/2
  Constant2/1 -> Manual Switch1/1
  Constant5/1 -> Manual Switch/1
  Constant6/1 -> Switch2/3
  Manual Switch1/1 -> [ReconfigSwitch]
  [error_switch_signal] -> Switch2/1
  [e_s_signal] -> IC4/1
  Decition Making/2 -> If Action Subsystem4/Action
  Matrizes A2/1 -> Subsystem1/2(C)
  iL Observer/1(x_hat) -> [x_hat_iL]
  Matrizes A1/1 -> [CVc]
  [CVc] -> Subsystem/2(C)
  Matrizes A3/1 -> [CiL]
  [CiL] -> iL Observer/1(C)
  [Clock] -> If Action Subsystem4/2(clock)
  [y_fault] -> IC8/1
  Step1/1 -> Manual Switch2/1
  [x_hat_iL] -> Scope4/1
  [y_fault] -> Scope5/1
  [sigma] -> Boost Converter/1(sigma)
  [alarmTrue] -> IC/1
  AntiFalseAlarm/1(FaultClass) -> [typeFaultIsolated]
  [x_hat_iL] -> Demux/1
  From51/1 -> Corrente_Il1/1, Scope19/1
  Demux/1 -> To Workspace14/1
  Demux1/2 -> To Workspace3/1
  [J] -> Tensão Vc6/1, Scope7/1
  [y_fault] -> Demux4/1
  From40/1 -> Scope24/2  "Sliding Mode"
  Demux4/2 -> To Workspace10/1
  Demux2/2 -> To Workspace6/1
  From48/1 -> Scope18/2  "Sliding Mode"
  [typeFaultIsolated] -> Scope6/1
  From35/1 -> Scope18/1  "Sensor"
  [alarm] -> Scope12/1
  [e_y] -> To Workspace8/1
  [f_s] -> To Workspace12/1
  [y_fault] -> Scope20/1
  [alarm] -> To Workspace11/1
  [e_s_signal] -> To Workspace13/1
  ? -> Scope/1, To Workspace18/1
  Demux2/1 -> To Workspace4/1
  From77/1 -> Scope13/1  "Sensorl"
  Demux1/1 -> To Workspace1/1
  [x] -> Scope21/1
  ? -> To Workspace9/1, Scope15/1
  From71/1 -> ?
  ? -> To Workspace5/1
  [x] -> Demux2/1
  From37/1 -> Tensão Vc14/1, Scope23/1
  From73/1 -> Scope8/2  "Real"
  From52/1 -> Scope14/1, Tensão Vc4/1  "Sliding Mode"
  [typeFaultIsolated] -> To Workspace2/1
  From42/1 -> Scope24/1  "Real"
  From69/1 -> Scope8/1  "Sensorl"
  [Clock] -> Display/1
  From49/1 -> Scope17/1, Tensão Vc5/1  "Sliding Mode"
  From60/1 -> Scope9/2  "Real"
  Demux/2 -> To Workspace16/1
  From57/1 -> Scope9/1  "Sensor"
  Demux4/1 -> To Workspace7/1
  From66/1 -> Scope22/1, Tensão Vc1/1
  [x_hat_Vc] -> Demux1/1
  From67/1 -> Scope11/1, Corrente_Il2/1
  [nnoutpu] -> To Workspace15/1
  [y_e_tilde] -> To Workspace17/1
  [J] -> To Workspace19/1
  Constant4/1 -> Fault Detecition/1
  Constant3/1 -> Fault Detecition/3
  Residual Generator2/1(RMS) -> Fault Detecition/2, [J]
  Fault Detecition/1 -> [alarmTrue]
  [v] -> Scope10/1
  [y_fault] -> Subsystem1/1(y)
  Vc OBserver/2(y_hat) -> IC2/1, [y_hat_Vc]
  [y_fault] -> Sum4/2, Subsystem9/1(x)
  Gain/1 -> [y]
  [y] -> D(f_s)/1(y)
  [xe] -> Gain1/1
  Gain1/1 -> Sum4/1
  ErrorGenerator/1(e_y) -> Sliding Mode Observer 5/1(ey)
  ErrorGenerator/2(v) -> Sliding Mode Observer 5/2(v), [v]
  [sigma] -> Sliding Mode Observer 5/3(sigma)
  Sliding Mode Observer 5/2(y_e_tilde_hat) -> IC1/1, [y_e_tilde_hat]
  Sliding Mode Observer 5/1(ey_out) -> [e_y]
  IC/1 -> AntiFalseAlarm/2(Alarm)
  Subsystem/1(error) -> [VcOBsErrror], Vc OBserver/1(ObserverError)
  Vc OBserver/1(x_hat) -> [x_hat_Vc]
  [sigma] -> iL Observer/3(sigma)
  Subsystem1/1(error) -> [iL_obs_error], iL Observer/2(ObserverError)
  [CVc] -> Vc OBserver/2(C)
  iL Observer/2(y_hat) -> IC3/1, [y_hat_iL]
  IC1/1 -> ErrorGenerator/2(y_e_tilde_hat)
  IC2/1 -> Subsystem/4(y_hat)
  IC3/1 -> Subsystem1/4(y_hat)
  IC4/1 -> Decition Making/1, Scope16/1
  IC5/1 -> If Action Subsystem/1(In1)
  [y_fault] -> IC5/1
  [x_hat_iL] -> IC6/1
  IC7/1 -> If Action Subsystem1/1(y)
  [x_hat_Vc] -> IC7/1
  IC8/1 -> If Action Subsystem3/1(In1)
  [e_y] -> IC9/1
  IC9/1 -> Residual Generator2/1(e_y)
  [x_reconfig] -> IC10/1
  IC10/1 -> Controlador1/2(x)
  AntiFalseAlarm/2(AlarmOut) -> [alarm]
  [alarmTrue] -> To Workspace20/1
  [Clock] -> If Action Subsystem1/2(clock)
  If Action Subsystem1/1(x_hat) -> Merge/3
  Decition Making/4 -> If Action Subsystem3/Action
  If Action Subsystem3/1(Out1) -> Merge/4
  If Action Subsystem/2(RESET) -> Merge1/1
  If Action Subsystem1/2(RESET) -> Merge1/2
  If Action Subsystem3/2(RESET) -> Merge1/4
  Merge1/1 -> [RESET]
  [RESET] -> IC11/1
  IC11/1 -> Subsystem/3(RESET)
  IC12/1 -> Subsystem1/3(RESET)
  IC6/1 -> If Action Subsystem4/1(y)
  If Action Subsystem4/1(x_hat) -> Merge/2
  If Action Subsystem4/2(RESET) -> Merge1/3
  [RESET] -> IC12/1
  [x_hat_Vc] -> Sum/1, Demux5/1
  [x_hat_iL] -> Sum/2, Demux6/1
  Demux5/1 -> Sum1/1
  Demux6/1 -> Sum1/2
  Demux5/2 -> Sum2/1
  Demux6/2 -> Sum2/2
  Sum2/1 -> [deltaVc], Residual Generator3/1(e_y)
  From24/1 -> Sum5/1, Sum3/1
  From27/1 -> Sum3/2
  From29/1 -> Sum5/2
  Sum5/1 -> Matrix Square2/1
  Sqrt2/1 -> Moving RMS/1
  Sum3/1 -> Matrix Square1/1
  Matrix Square1/1 -> Sum6/1
  Matrix Square2/1 -> Sum6/2
  Sum6/1 -> Sqrt2/1
  Moving RMS/1 -> Sqrt1/1
  Sqrt1/1 -> Scope26/1
  Fault Identification Neural Netowrk/1(netOutputs) -> AntiFalseAlarm/1(PRNN), Scope27/1, [nnoutpu]
  Sum1/1 -> [deltaiL]
  [deltaVc] -> Mux2/3
  [deltaiL] -> Mux2/2

== system boostObserver_old/Subsystem/AntiFalseAlarm ==
  PRNN : Inport
  Alarm : Inport  Port=2
  Constant7 : Constant
  FaultDetecition1 : Switch  Criteria=u2 > Threshold
  Product1 : Product
  Step1 : Step  Time=AlarmDeadTime  SampleTime=0
  FaultClass : Outport
  AlarmOut : Outport  Port=2
  wires:
  PRNN/1 -> FaultDetecition1/1
  Constant7/1 -> FaultDetecition1/3
  Step1/1 -> Product1/1
  Alarm/1 -> Product1/2
  FaultDetecition1/1 -> FaultClass/1
  Product1/1 -> AlarmOut/1, FaultDetecition1/2

== system boostObserver_old/Subsystem/Augmented Error Generator ==
  e : Inport
  Mux : Mux  Inputs=2
  z1 : Subsystem
  e_tilde : Outport
  wires:
  z1/1(z) -> Mux/2
  Mux/1 -> e_tilde/1
  e/1 -> Mux/1, z1/1(z_dot)

== system boostObserver_old/Subsystem/Boost Converter ==
  note: Escolha do tipo de entrada
  note: Circuito do conversor
  sigma : Inport
  ConversorBoost : Subsystem
  Mux1 : Mux  Inputs=2
  Terminator : Terminator
  Terminator1 : Terminator
  TipoEntrada : Subsystem
  x : Outport
  wires:
  TipoEntrada/4("Rvariavel ") -> [Rinput]
  sigma/1 -> ConversorBoost/1(sigma)
  [Vinput1] -> ConversorBoost/2(Vinput1)
  [Vinput2] -> ConversorBoost/3(Vinput2)
  [Rinput] -> ConversorBoost/5(Rinput)
  TipoEntrada/5("Rparallelvariavel ") -> [Rparallelinput]
  [Rparallelinput] -> ConversorBoost/6(Rparallelinput)
  [Vinput3] -> ConversorBoost/4(Vinput3)
  TipoEntrada/1(Vu) -> [Vinput1]
  TipoEntrada/2(VuAdd) -> [Vinput2]
  TipoEntrada/3(VuRemove) -> [Vinput3]
  ConversorBoost/1(iLoutput) -> Mux1/1
  ConversorBoost/2(Vcoutput) -> Mux1/2
  Mux1/1 -> x/1
  ConversorBoost/3(iro) -> Terminator/1
  ConversorBoost/4(Vu) -> Terminator1/1

== system boostObserver_old/Subsystem/Controlador1 ==
  note: Sinal de controle
  note: Superfície
  note: Ponto de equilíbrio
  ve : Inport
  x : Inport  Port=2
  "    " : Constant  Value=ueq
  "    2" : Constant  Value=Smep
  Constant6 : Constant  Value=boost_parameters
  Demux1 : Demux  Outputs=2
  Demux2 : Demux  Outputs=2
  Gain : Gain  Gain=0.8
  Gain1 : Gain  Gain=8
  Gain3 : Gain  Gain=2.3
  Integrator1 : Integrator
  PWM : powerlib_meascontrol/Pulse & Signal Generators/PWM Generator (DC-DC)  Fsw=7000  Ts=0
  Scope : Scope
  SlidingSurface : Subsystem
  Sum : Sum  Inputs=|++
  Sum4 : Sum  Inputs=++|
  Sum5 : Sum  Inputs=-+|
  Sum6 : Sum  Inputs=-+|
  Sum9 : Sum  Inputs=|++
  xe : MATLAB Function  TreatAsAtomicUnit=on
  sigma : Outport
  i_e : Outport  Port=2
  x_e : Outport  Port=3
  wires:
  Demux1/1 -> Sum6/2  "IL"
  PWM/1 -> sigma/1
  ve/1 -> xe/2(ve)
  Demux2/2 -> Sum5/1  "Vo1"
  "    "/1 -> Sum9/2
  Sum5/1 -> Gain3/1, Gain/1
  Sum9/1 -> PWM/1
  Demux1/2 -> Sum5/2  "Vo1"
  Demux2/1 -> Sum6/1
  xe/2(i_e) -> i_e/1
  x/1 -> Demux2/1
  Constant6/1 -> xe/1(boost_parameters)
  Gain1/1 -> Sum4/2
  xe/1(x_e) -> Demux1/1, x_e/1
  Gain/1 -> Sum/1
  Sum/1 -> Sum4/1
  SlidingSurface/1(d) -> Scope/1, Sum9/1
  "    2"/1 -> SlidingSurface/2(ep)
  Sum6/1 -> Gain1/1
  Gain3/1 -> Integrator1/1
  Integrator1/1 -> Sum/2
  Sum4/1 -> SlidingSurface/1(S)

== system boostObserver_old/Subsystem/D(f_s) ==
  note: iL Sensor Faults
  note: Vc Sensor Faults
  y : Inport
  Constant1 : Constant  Value=VcFaultSwitch
  Constant2 : Constant  Value=iLGainFaultFactor
  Constant3 : Constant  Value=VcNoiseFaultSwitch
  Constant4 : Constant  Value=VcGainFaultFactor
  Constant7 : Constant  Value=iLFaultSwitch
  Constant8 : Constant  Value=iLNoiseFaultSwitch
  Demux : Demux  Outputs=2
  Mux : Mux  Inputs=2
  Step10 : Step  Time=VcFaultTime  SampleTime=0
  Step2 : Step  Time=VcNoiseTime  SampleTime=0
  Step8 : Step  Time=iLFaultTime  SampleTime=0
  Step9 : Step  Time=iLNoiseTime  SampleTime=0
  Subsystem : Subsystem
  Subsystem2 : Subsystem
  Sum : Sum  Inputs=|+-
  y_fault : Outport
  wires:
  [iLoutput] -> Subsystem/1(input)
  Constant7/1 -> Subsystem/4(FaultSwtich)
  Constant8/1 -> Subsystem/5(NoiseFaultSwitch)
  Step8/1 -> Subsystem/2(FaultStep)
  Step9/1 -> Subsystem/3(NoiseStep)
  Constant1/1 -> Subsystem2/4(FaultSwtich)
  Constant3/1 -> Subsystem2/5(NoiseFaultSwitch)
  Step10/1 -> Subsystem2/2(FaultStep)
  Step2/1 -> Subsystem2/3(NoiseStep)
  Constant2/1 -> Subsystem/6(FaultFactor)
  Constant4/1 -> Subsystem2/6(FaultFactor)
  [VcOutput] -> Subsystem2/1(input)
  Demux/1 -> [iLoutput]
  Demux/2 -> [VcOutput]
  y/1 -> [y], Demux/1
  Subsystem/1(output) -> Mux/1
  Subsystem2/1(output) -> Mux/2
  Mux/1 -> Sum/2, y_fault/1
  [y] -> Sum/1

== system boostObserver_old/Subsystem/ErrorGenerator ==
  y_e_tilde : Inport
  y_e_tilde_hat : Inport  Port=2
  AND : Logic  IconShape=distinctive  AllPortsSameDT=off  OutDataTypeStr=boolean
  Compare To Zero : simulink/Logic and Bit Operations/Compare To Zero  relop=~=  OutDataTypeStr=boolean
  Constant1 : Constant  Value=[0;0]
  Demux : Demux  Outputs=2
  If : If  IfExpression=u1 ~= 0
  If Action Subsystem : Subsystem  TreatAsAtomicUnit=on
  If Action Subsystem1 : Subsystem  TreatAsAtomicUnit=on
  Merge : Merge  InitialOutput=[0;0]
  Sum : Sum  Inputs=|+-
  e_y : Outport
  v : Outport  Port=2
  wires:
  y_e_tilde/1 -> Sum/1
  y_e_tilde_hat/1 -> Sum/2
  Sum/1 -> Compare To Zero/1, e_y/1, [e_y]
  If/1 -> If Action Subsystem/Action
  If/2 -> If Action Subsystem1/Action
  [e_y] -> If Action Subsystem/1(e_y)
  Constant1/1 -> If Action Subsystem1/1(e_y)
  If Action Subsystem/1(v) -> Merge/1
  If Action Subsystem1/1(v) -> Merge/2
  Demux/1 -> AND/1
  Demux/2 -> AND/2
  AND/1 -> If/1
  Merge/1 -> v/1
  Compare To Zero/1 -> Demux/1
